simulink model "PWM2010a_TestPLL_fcut3"  (R2019b)
settings: Solver=VariableStepAuto  StartTime=0.0  StopTime=1  RelTol=1e-3
InitFcn:
  | fcut=20;fpi=5;Vm=310;
  | fbase=50;
  | Kp=fcut/Vm;
  | Ki=2*pi*fpi*Kp;
libraries: powerlib_extras x1
settings Model: Creator=W002220B  LastModifiedBy=W002220B

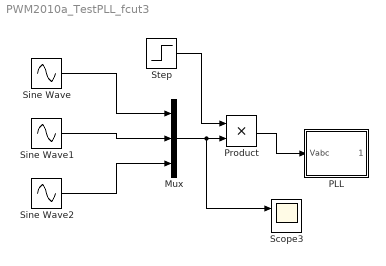
== system PWM2010a_TestPLL_fcut3 ==
  Mux : Mux  Inputs=3
  PLL : Subsystem
  Product : Product
  Scope3 : Scope  NumInputPorts=2
  Sine Wave : Sin  Amplitude=310  Frequency=50*2*pi  Phase=pi/2  SampleTime=0
  Sine Wave1 : Sin  Amplitude=310  Frequency=50*2*pi  Phase=pi/2-2*pi/3  SampleTime=0
  Sine Wave2 : Sin  Amplitude=310  Frequency=50*2*pi  Phase=pi/2+2*pi/3  SampleTime=0
  Step : Step  Time=0.5  Before=1  SampleTime=0
  wires:
  Mux/1 -> Scope3/1, Product/2
  Product/1 -> PLL/1(Vabc)
  Step/1 -> Product/1
  Sine Wave1/1 -> Mux/2
  Sine Wave/1 -> Mux/1
  Sine Wave2/1 -> Mux/3

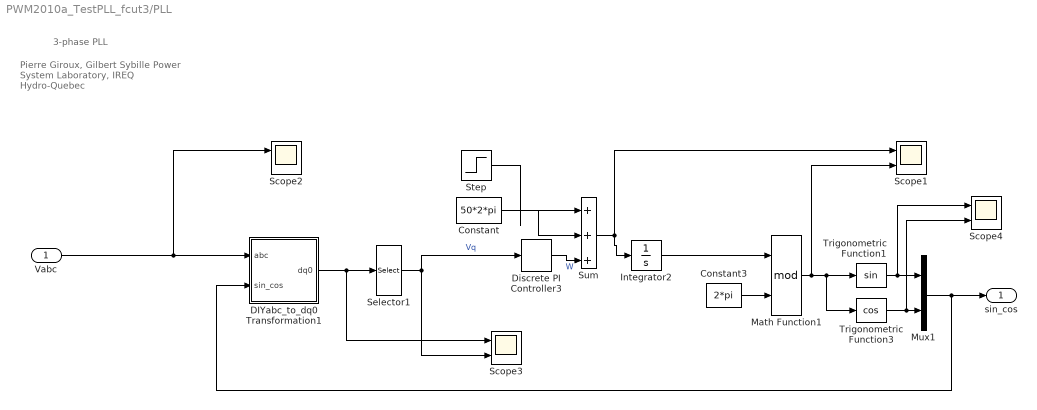
== system PWM2010a_TestPLL_fcut3/PLL ==
  note: 3-phase PLL
  note: Pierre Giroux, Gilbert Sybille
      | Power System Laboratory, IREQ
      | Hydro-Quebec
  Vabc : Inport  PortDimensions=3
  Constant : Constant  Value=50*2*pi
  Constant3 : Constant  Value=2*pi
  DIYabc_to_dq0 Transformation1 : Subsystem  AncestorBlock=powerlib_extras/Measurements/abc_to_dq0 Transformation  mask(abc to dq0 Transformation){}
      mask help:
      | This block performs the  abc to dq0 transformation on a set of three-phase signals. It computes the direct axis Vd, quadratic axis Vq, and zero sequence V0 quantities in a two axis rotating reference frame according to the following transformation:
      |
      |
      | Vd = 2/3*[Va*cos(wt) + Vb*cos(wt-2pi/3) + Vc*cos(wt+2pi/3)]
      | Vq = 2/3*[-Va*sin(wt) - Vb*sin(wt-2pi/3) - Vc*sin(wt+2pi/3)]
      | V0 = 1/3*[Va +  Vb  +  Vc ]
      |
      | where w=  rotation speed (rad/s) of the rotating frame.
      |
      | This transformation is commonly used in three-phase electric machine models where it is known as the Park transformation.
      mask Help: web(psbhelp);
  Discrete PI Controller3 : powerlib_extras/Discrete  Control Blocks/Discrete PI Controller  Kp=Kp  Ki=Ki  Par_Limits=[1e6 -1e6]  Init=0  Ts=50e-6
      settings: SourceProductName=Simscape Electrical
  Integrator2 : Integrator
  Math Function1 : Math  Operator=mod  SaturateOnIntegerOverflow=on
  Mux1 : Mux  Inputs=2
  Scope{1..4} (4 alike) : Scope  NumInputPorts=2
  Selector1 : Selector  InputPortWidth=3  IndexOptions=Index vector (dialog)  Indices=2  OutputSizes=1
  Step : Step  Time=0.5  After=-25*2*pi  SampleTime=0
  Sum : Sum  Inputs=|+++
  Trigonometric Function1 : Trigonometry
  Trigonometric Function3 : Trigonometry  Operator=cos
  sin_cos : Outport
  wires:
  Vabc/1 -> Scope2/1, DIYabc_to_dq0 Transformation1/1(abc)
  DIYabc_to_dq0 Transformation1/1(dq0) -> Selector1/1, Scope3/1
  Constant3/1 -> Math Function1/2
  Math Function1/1 -> Scope1/2, Trigonometric Function1/1, Trigonometric Function3/1
  Trigonometric Function1/1 -> Scope4/1, Mux1/1
  Trigonometric Function3/1 -> Scope4/2, Mux1/2
  Mux1/1 -> sin_cos/1, DIYabc_to_dq0 Transformation1/2(sin_cos)
  Selector1/1 -> Scope3/2, Discrete PI Controller3/1  "Vq"
  Integrator2/1 -> Math Function1/1
  Sum/1 -> Integrator2/1, Scope1/1
  Discrete PI Controller3/1 -> Sum/3  "W"
  Constant/1 -> Sum/2
  Step/1 -> Sum/1

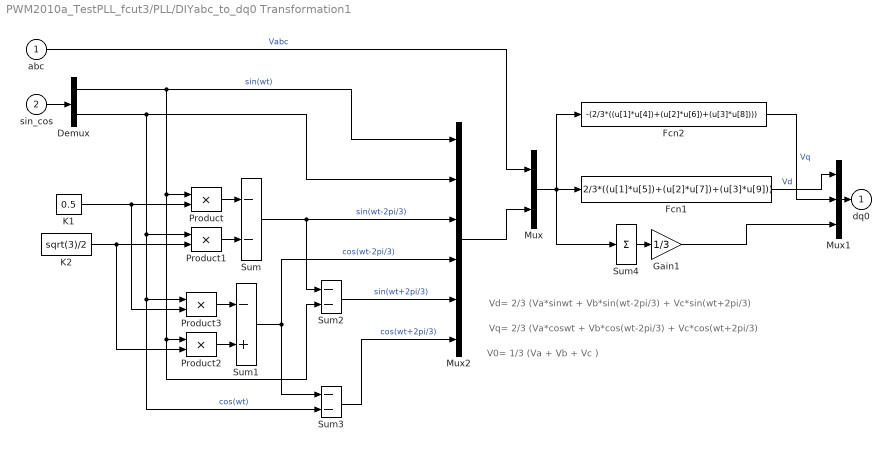
== system PWM2010a_TestPLL_fcut3/PLL/DIYabc_to_dq0 Transformation1 ==
  note: V0= 1/3 (Va + Vb + Vc )
  note: Vd= 2/3 (Va*sinwt + Vb*sin(wt-2pi/3) + Vc*sin(wt+2pi/3)
  note: Vq= 2/3 (Va*coswt + Vb*cos(wt-2pi/3) + Vc*cos(wt+2pi/3)
  abc : Inport  PortDimensions=3
  sin_cos : Inport  Port=2  PortDimensions=2
  Demux : Demux  Outputs=2
  Fcn1 : Fcn  Expr=2/3*((u[1]*u[5])+(u[2]*u[7])+(u[3]*u[9]))
  Fcn2 : Fcn  Expr=-(2/3*((u[1]*u[4])+(u[2]*u[6])+(u[3]*u[8])))
  Gain1 : Gain  Gain=1/3  SaturateOnIntegerOverflow=on  OutDataTypeStr=Inherit: Same as input  ParamDataTypeStr=Inherit: Same as input
  K1 : Constant  Value=0.5
  K2 : Constant  Value=sqrt(3)/2
  Mux : Mux  Inputs=2
  Mux1 : Mux  Inputs=3
  Mux2 : Mux  Inputs=6
  Product{,1..3} (4 alike) : Product  SaturateOnIntegerOverflow=on  InputSameDT=on  OutDataTypeStr=Inherit: Same as first input
  Sum : Sum  Inputs=--  SaturateOnIntegerOverflow=on  InputSameDT=on  OutDataTypeStr=Inherit: Same as first input
  Sum1 : Sum  Inputs=-+  SaturateOnIntegerOverflow=on  InputSameDT=on  OutDataTypeStr=Inherit: Same as first input
  Sum2 : Sum  Inputs=--  SaturateOnIntegerOverflow=on  InputSameDT=on  OutDataTypeStr=Inherit: Same as first input
  Sum3 : Sum  Inputs=--  SaturateOnIntegerOverflow=on  InputSameDT=on  OutDataTypeStr=Inherit: Same as first input
  Sum4 : Sum  Inputs=1  SaturateOnIntegerOverflow=on  InputSameDT=on  OutDataTypeStr=Inherit: Same as first input
  dq0 : Outport  InitialOutput=0
  wires:
  Fcn1/1 -> Mux1/1  "Vd"
  Fcn2/1 -> Mux1/2  "Vq"
  Mux1/1 -> dq0/1
  Sum4/1 -> Gain1/1
  Mux/1 -> Sum4/1, Fcn1/1, Fcn2/1
  Sum1/1 -> Sum3/1, Mux2/4  "cos(wt-2pi/3)"
  Sum/1 -> Sum2/1, Mux2/3  "sin(wt-2pi/3)"
  K2/1 -> Product2/2, Product1/2
  K1/1 -> Product3/2, Product/2
  Sum2/1 -> Mux2/5  "sin(wt+2pi/3)"
  Sum3/1 -> Mux2/6  "cos(wt+2pi/3)"
  Product2/1 -> Sum1/2
  Product3/1 -> Sum1/1
  Product1/1 -> Sum/2
  Product/1 -> Sum/1
  Demux/1 -> Mux2/1, Sum2/2, Product2/1, Product/1  "sin(wt)"
  Demux/2 -> Mux2/2, Product1/1, Product3/1, Sum3/2  "cos(wt)"
  sin_cos/1 -> Demux/1
  Mux2/1 -> Mux/2
  abc/1 -> Mux/1  "Vabc"
  Gain1/1 -> Mux1/3
